simulink model "LQR_nonlinear_sim"  (R2025b)
settings: Solver=VariableStepAuto  StartTime=0.0  StopTime=5  RelTol=1e-3
undefined symbols (not defined in the file): A, B, bb, C, D, dotphi_x_ref, dotphi_y_ref, ic, ic_xy, ic_xz, ic_yz, K, K_vert, K_xy, Kr, N_vert
settings Model: Creator=JPham  LastModifiedBy=JPham

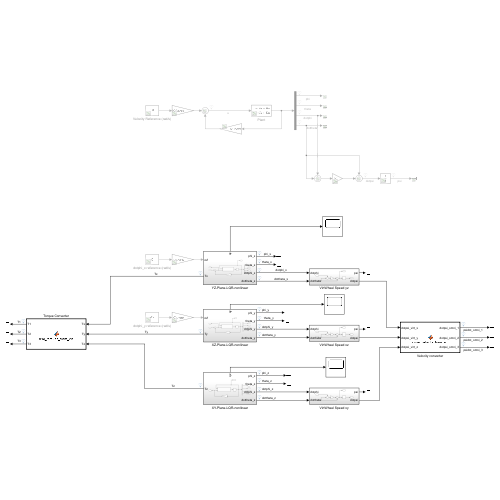
[thumbnail: Simulink's stored preview of the top-level diagram]
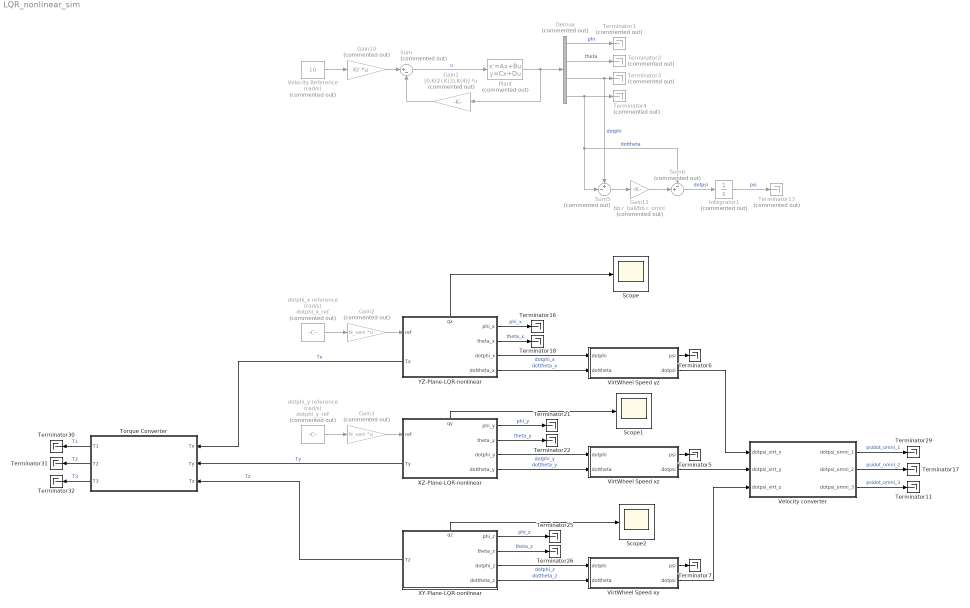
== system LQR_nonlinear_sim ==
  Demux : Demux  Commented=on
  Gain1 : Gain  Commented=on  Gain=[0,K(2),K(3),K(4)]  Multiplication=Matrix(K*u) (u vector)
  Gain10 : Gain  Commented=on  Gain=Kr  Multiplication=Matrix(K*u) (u vector)
  Gain11 : Gain  Commented=on  Gain=bb.r_ball/bb.r_omni
  Gain2 : Gain  Commented=on  Gain=N_vert  Multiplication=Matrix(K*u) (u vector)
  Gain3 : Gain  Commented=on  Gain=N_vert  Multiplication=Matrix(K*u) (u vector)
  Integrator1 : Integrator  Commented=on
  Plant : StateSpace  Commented=on  A=A  B=B  C=C  D=D  InitialCondition=ic  ContinuousStateAttributes={'phi', 'theta', 'dot_phi', 'dot_theta'}
  Scope : Scope
      settings: ActiveDisplayYMinimum=-1  ActiveDisplayYMaximum=1
  Scope1 : Scope
  Scope2 : Scope
      settings: DataLoggingVariableName=ScopeData2
  Sum : Sum  Commented=on  Inputs=|+-
  Sum5 : Sum  Commented=on  Inputs=+-|
  Sum6 : Sum  Commented=on  Inputs=-+|
  Terminator{1..4,13} (5 alike) : Terminator  Commented=on
  Terminator{5..7,11,16..18,21..22,25..26,29..32} (15 alike) : Terminator
  Torque Converter : MATLAB Function  TreatAsAtomicUnit=on
  Velocity Reference (rad/s) : Constant  Commented=on  Value=10
  Velocity converter : MATLAB Function  TreatAsAtomicUnit=on
  VirtWheel Speed xy : Subsystem
  VirtWheel Speed xz : Subsystem
  VirtWheel Speed yz : Subsystem
  XY-Plane-LQR-nonlinear : Subsystem
      settings: PortSchema="{\"entries\":[{\"content\":{\"sides\":[{\"content\":{\"connectorIds\":[\"Out6\"]},\"type\":\"ConnectorPlacement.EquallySpacedRectSide\",\"uuid\":\"02b8159c-179d-4bec-803c-aa283f49b9c0\"},{\"content\":{\"connectorIds\":[\"Out1\",\"Out2\",\"Out3\",\"Out4\"],\"side\":\"RIGHT\"},\"type\":\"ConnectorPlacement.EquallySpacedRectSide\",\"uuid\":\"3221cdc4-2dbb-4803-8373-e56db730aa56\"},{\"content\":{\"connectorIds\":[\"Out5\"],\"side\":\"TOP\"},\"type\":\"ConnectorPlacement.EquallySpacedRectSide\",\"uuid\":\"2bc7cb91-f8b8-434b-9ab0-3d8179530137\"}]},\"type\":\"ConnectorPlacement.EquallySpacedConnector\",\"uuid\":\"c9142ecd-3781-401c-ba0b-68be917d9976\"}],\"packageUris\":[\"http://schema.mathworks.com/mf0/Connector/R2020b\"],\"version\":\"1.0\"}"
  XZ-Plane-LQR-nonlinear : Subsystem
      settings: PortSchema="{\"entries\":[{\"content\":{\"sides\":[{\"content\":{\"connectorIds\":[\"In1\",\"Out6\"]},\"type\":\"ConnectorPlacement.EquallySpacedRectSide\",\"uuid\":\"02b8159c-179d-4bec-803c-aa283f49b9c0\"},{\"content\":{\"connectorIds\":[\"Out1\",\"Out2\",\"Out3\",\"Out4\"],\"side\":\"RIGHT\"},\"type\":\"ConnectorPlacement.EquallySpacedRectSide\",\"uuid\":\"3221cdc4-2dbb-4803-8373-e56db730aa56\"},{\"content\":{\"connectorIds\":[\"Out5\"],\"side\":\"TOP\"},\"type\":\"ConnectorPlacement.EquallySpacedRectSide\",\"uuid\":\"2bc7cb91-f8b8-434b-9ab0-3d8179530137\"}]},\"type\":\"ConnectorPlacement.EquallySpacedConnector\",\"uuid\":\"c9142ecd-3781-401c-ba0b-68be917d9976\"}],\"packageUris\":[\"http://schema.mathworks.com/mf0/Connector/R2020b\"],\"version\":\"1.0\"}"
  YZ-Plane-LQR-nonlinear : Subsystem
      settings: PortSchema="{\"entries\":[{\"content\":{\"sides\":[{\"content\":{\"connectorIds\":[\"In1\",\"Out6\"]},\"type\":\"ConnectorPlacement.EquallySpacedRectSide\",\"uuid\":\"02b8159c-179d-4bec-803c-aa283f49b9c0\"},{\"content\":{\"connectorIds\":[\"Out1\",\"Out2\",\"Out3\",\"Out4\"],\"side\":\"RIGHT\"},\"type\":\"ConnectorPlacement.EquallySpacedRectSide\",\"uuid\":\"3221cdc4-2dbb-4803-8373-e56db730aa56\"},{\"content\":{\"connectorIds\":[\"Out5\"],\"side\":\"TOP\"},\"type\":\"ConnectorPlacement.EquallySpacedRectSide\",\"uuid\":\"2bc7cb91-f8b8-434b-9ab0-3d8179530137\"}]},\"type\":\"ConnectorPlacement.EquallySpacedConnector\",\"uuid\":\"c9142ecd-3781-401c-ba0b-68be917d9976\"}],\"packageUris\":[\"http://schema.mathworks.com/mf0/Connector/R2020b\"],\"version\":\"1.0\"}"
  dotphi_x reference (rad/s) : Constant  Commented=on  Value=dotphi_x_ref
  dotphi_y reference (rad/s) : Constant  Commented=on  Value=dotphi_y_ref
  wires:
  Velocity Reference (rad/s)/1 -> Gain10/1
  Demux/1 -> Terminator1/1  "phi"
  Sum5/1 -> Gain11/1
  Sum6/1 -> Integrator1/1  "dotpsi"
  Demux/3 -> Sum5/1, Terminator3/1  "dotphi"
  Integrator1/1 -> Terminator13/1  "psi"
  Demux/2 -> Terminator2/1  "theta"
  Demux/4 -> Terminator4/1, Sum5/2, Sum6/1  "dottheta"
  Plant/1 -> Gain1/1, Demux/1
  Gain11/1 -> Sum6/2
  Gain10/1 -> Sum/1
  Sum/1 -> Plant/1  "u"
  Gain1/1 -> Sum/2
  VirtWheel Speed yz/2(dotpsi) -> Velocity converter/1(dotpsi_virt_x)
  VirtWheel Speed xy/2(dotpsi) -> Velocity converter/3(dotpsi_virt_z)
  Torque Converter/3(T3) -> Terminator32/1  "T3"
  Torque Converter/2(T2) -> Terminator31/1  "T2"
  Torque Converter/1(T1) -> Terminator30/1  "T1"
  VirtWheel Speed xz/2(dotpsi) -> Velocity converter/2(dotpsi_virt_y)
  VirtWheel Speed xz/1(psi) -> Terminator5/1
  VirtWheel Speed yz/1(psi) -> Terminator6/1
  VirtWheel Speed xy/1(psi) -> Terminator7/1
  YZ-Plane-LQR-nonlinear/6(Tx) -> Torque Converter/1(Tx)  "Tx"
  XZ-Plane-LQR-nonlinear/6(Ty) -> Torque Converter/2(Ty)  "Ty"
  XY-Plane-LQR-nonlinear/6(Tz) -> Torque Converter/3(Tz)  "Tz"
  YZ-Plane-LQR-nonlinear/3(dotphi_x) -> VirtWheel Speed yz/1(dotphi)  "dotphi_x"
  YZ-Plane-LQR-nonlinear/4(dottheta_x) -> VirtWheel Speed yz/2(dottheta)  "dottheta_x"
  YZ-Plane-LQR-nonlinear/2(theta_x) -> Terminator18/1  "theta_x"
  YZ-Plane-LQR-nonlinear/1(phi_x) -> Terminator16/1  "phi_x"
  XZ-Plane-LQR-nonlinear/4(dottheta_y) -> VirtWheel Speed xz/2(dottheta)  "dottheta_y"
  XZ-Plane-LQR-nonlinear/1(phi_y) -> Terminator21/1  "phi_y"
  XZ-Plane-LQR-nonlinear/2(theta_y) -> Terminator22/1  "theta_y"
  XZ-Plane-LQR-nonlinear/3(dotphi_y) -> VirtWheel Speed xz/1(dotphi)  "dotphi_y"
  XY-Plane-LQR-nonlinear/4(dottheta_z) -> VirtWheel Speed xy/2(dottheta)  "dottheta_z"
  XY-Plane-LQR-nonlinear/1(phi_z) -> Terminator25/1  "phi_z"
  XY-Plane-LQR-nonlinear/2(theta_z) -> Terminator26/1  "theta_z"
  XY-Plane-LQR-nonlinear/3(dotphi_z) -> VirtWheel Speed xy/1(dotphi)  "dotphi_z"
  dotphi_x reference (rad/s)/1 -> Gain2/1
  Gain2/1 -> YZ-Plane-LQR-nonlinear/1(ref)
  dotphi_y reference (rad/s)/1 -> Gain3/1
  Gain3/1 -> XZ-Plane-LQR-nonlinear/1(ref)
  Velocity converter/2(dotpsi_omni_2) -> Terminator17/1  "psidot_omni_2"
  Velocity converter/1(dotpsi_omni_1) -> Terminator29/1  "psidot_omni_1"
  Velocity converter/3(dotpsi_omni_3) -> Terminator11/1  "psidot_omni_3"
  YZ-Plane-LQR-nonlinear/5(qx) -> Scope/1
  XZ-Plane-LQR-nonlinear/5(qy) -> Scope1/1
  XY-Plane-LQR-nonlinear/5(qz) -> Scope2/1

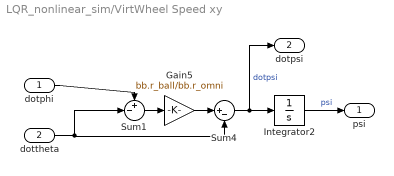
== system LQR_nonlinear_sim/VirtWheel Speed xy ==
  dotphi : Inport
  dottheta : Inport  Port=2
  Gain5 : Gain  Gain=bb.r_ball/bb.r_omni
  Integrator2 : Integrator
  Sum1 : Sum  Inputs=+-|
  Sum4 : Sum  Inputs=|+-
  psi : Outport
  dotpsi : Outport  Port=2
  wires:
  Sum1/1 -> Gain5/1
  dotphi/1 -> Sum1/1
  Integrator2/1 -> psi/1  "psi"
  Sum4/1 -> Integrator2/1, dotpsi/1  "dotpsi"
  dottheta/1 -> Sum4/2, Sum1/2
  Gain5/1 -> Sum4/1

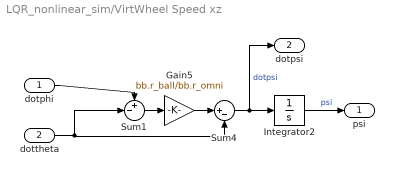
== system LQR_nonlinear_sim/VirtWheel Speed xz ==
  dotphi : Inport
  dottheta : Inport  Port=2
  Gain5 : Gain  Gain=bb.r_ball/bb.r_omni
  Integrator2 : Integrator
  Sum1 : Sum  Inputs=+-|
  Sum4 : Sum  Inputs=|+-
  psi : Outport
  dotpsi : Outport  Port=2
  wires:
  Gain5/1 -> Sum4/1
  dottheta/1 -> Sum1/2, Sum4/2
  Sum4/1 -> dotpsi/1, Integrator2/1  "dotpsi"
  Integrator2/1 -> psi/1  "psi"
  dotphi/1 -> Sum1/1
  Sum1/1 -> Gain5/1

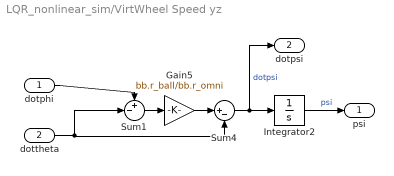
== system LQR_nonlinear_sim/VirtWheel Speed yz ==
  dotphi : Inport
  dottheta : Inport  Port=2
  Gain5 : Gain  Gain=bb.r_ball/bb.r_omni
  Integrator2 : Integrator
  Sum1 : Sum  Inputs=+-|
  Sum4 : Sum  Inputs=|+-
  psi : Outport
  dotpsi : Outport  Port=2
  wires:
  Sum1/1 -> Gain5/1
  dotphi/1 -> Sum1/1
  Integrator2/1 -> psi/1  "psi"
  Sum4/1 -> Integrator2/1, dotpsi/1  "dotpsi"
  dottheta/1 -> Sum4/2, Sum1/2
  Gain5/1 -> Sum4/1

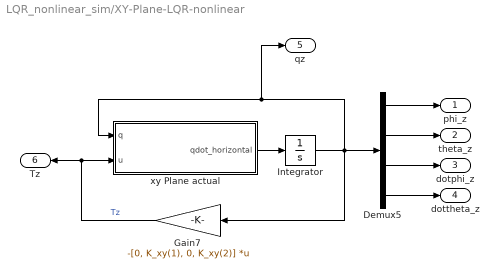
== system LQR_nonlinear_sim/XY-Plane-LQR-nonlinear ==
  Demux5 : Demux
  Gain7 : Gain  Gain=-[0, K_xy(1), 0, K_xy(2)]  Multiplication=Matrix(K*u) (u vector)
  Integrator : Integrator  InitialCondition=[0; ic_xy(1); 0; ic_xy(2)]
  xy Plane actual : MATLAB Function  TreatAsAtomicUnit=on
  phi_z : Outport
  theta_z : Outport  Port=2
  dotphi_z : Outport  Port=3
  dottheta_z : Outport  Port=4
  qz : Outport  Port=5
  Tz : Outport  Port=6
  wires:
  Demux5/1 -> phi_z/1
  Demux5/2 -> theta_z/1
  Integrator/1 -> qz/1, xy Plane actual/1(q), Gain7/1, Demux5/1
  Gain7/1 -> Tz/1, xy Plane actual/2(u)  "Tz"
  xy Plane actual/1(qdot_horizontal) -> Integrator/1
  Demux5/3 -> dotphi_z/1
  Demux5/4 -> dottheta_z/1

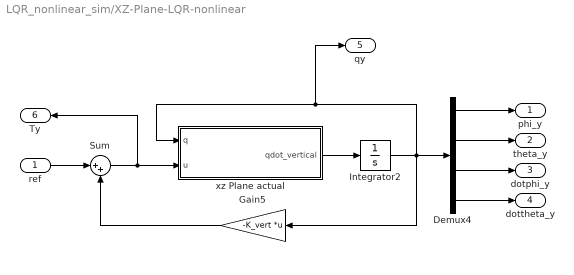
== system LQR_nonlinear_sim/XZ-Plane-LQR-nonlinear ==
  ref : Inport
  Demux4 : Demux
  Gain5 : Gain  Gain=-K_vert  Multiplication=Matrix(K*u) (u vector)
  Integrator2 : Integrator  InitialCondition=ic_xz  ContinuousStateAttributes='angle'
  Sum : Sum  Inputs=|++
  xz Plane actual : MATLAB Function  TreatAsAtomicUnit=on
  phi_y : Outport
  theta_y : Outport  Port=2
  dotphi_y : Outport  Port=3
  dottheta_y : Outport  Port=4
  qy : Outport  Port=5
  Ty : Outport  Port=6
  wires:
  Demux4/2 -> theta_y/1
  Integrator2/1 -> qy/1, xz Plane actual/1(q), Demux4/1, Gain5/1
  xz Plane actual/1(qdot_vertical) -> Integrator2/1
  Gain5/1 -> Sum/2
  Demux4/3 -> dotphi_y/1
  Demux4/1 -> phi_y/1
  Demux4/4 -> dottheta_y/1
  ref/1 -> Sum/1
  Sum/1 -> Ty/1, xz Plane actual/2(u)

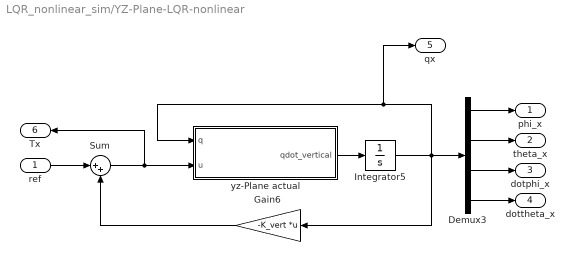
== system LQR_nonlinear_sim/YZ-Plane-LQR-nonlinear ==
  ref : Inport
  Demux3 : Demux
  Gain6 : Gain  Gain=-K_vert  Multiplication=Matrix(K*u) (u vector)
  Integrator5 : Integrator  InitialCondition=ic_yz  ContinuousStateAttributes='angle'
  Sum : Sum  Inputs=|++
  yz-Plane actual : MATLAB Function  TreatAsAtomicUnit=on
  phi_x : Outport
  theta_x : Outport  Port=2
  dotphi_x : Outport  Port=3
  dottheta_x : Outport  Port=4
  qx : Outport  Port=5
  Tx : Outport  Port=6
  wires:
  yz-Plane actual/1(qdot_vertical) -> Integrator5/1
  Integrator5/1 -> Gain6/1, Demux3/1, qx/1, yz-Plane actual/1(q)
  Demux3/3 -> dotphi_x/1
  Demux3/4 -> dottheta_x/1
  Gain6/1 -> Sum/2
  Demux3/2 -> theta_x/1
  Demux3/1 -> phi_x/1
  Sum/1 -> yz-Plane actual/2(u), Tx/1
  ref/1 -> Sum/1

== matlab function LQR_nonlinear_sim/YZ-Plane-LQR-nonlinear/yz-Plane actual ==
  data: q input; u input; qdot_vertical output
function qdot_vertical = f(q, u)
    % Define dimensions for code generation
    % x is 4x1 state: [phi; theta; phi_dot; theta_dot]
    % u is scalar torque (leave as constant for now)
    % p is the parameter structure, loaded into simulink in Model Explorer
    
    phi     = q(1); % phi
    theta   = q(2); % theta
    dotphi  = q(3); % phi_dot
    dottheta= q(4); % theta_dot
    
    p = params;
    % Aux Parameters
    m_tot = p.m_ball + p.m_body + p.m_virt;
    r_tot = p.r_ball + p.r_omni;
    gamma = p.l*p.m_body + (p.r_ball + p.r_omni)*p.m_virt;
    
    % M matrix
    M11 = m_tot * p.r_ball^2 + p.Theta_ball + (p.r_ball / p.r_omni)^2 * p.Theta_virt_vertical;
    M12 = -(p.r_ball / p.r_omni^2) * r_tot * p.Theta_virt_vertical + gamma * p.r_ball*cos(theta); 
    M22 = (r_tot^2 / p.r_omni^2) * p.Theta_virt_vertical + p.Theta_body_vertical + ...
           p.m_body * p.l^2 + p.m_virt * r_tot^2;
    M21 = M12;

    M = [M11, M12;
         M21, M22];
    
    % C vector
    Cvec = [ -p.r_ball*gamma*sin(theta)*dottheta^2; 
              0 ];
    % G vector
    Gvec = [ 0; 
            -p.g*sin(theta)*gamma ];
    % S vector (f_NP = S*u(t))
    S = [ p.r_ball / p.r_omni; -p.r_ball / p.r_omni ];
    
    % --- Dynamics Calculation ---
    F_np = S * u; 
    
    % Solve for qdd from M * qdd + C + G = F_np
    % qddot = M \ (F_np - C - G) = [theta_doubledot; phi_doubledot]
    qddot = M \ (F_np - Cvec - Gvec);
    
    % Assemble qdot_vertical
    qdot_vertical = [dotphi;
                     dottheta;
                     qddot(1);
                     qddot(2)];
end

== matlab function LQR_nonlinear_sim/XZ-Plane-LQR-nonlinear/xz Plane actual ==
  data: q input; u input; qdot_vertical output
function qdot_vertical = f(q, u)
    % Define dimensions for code generation
    % x is 4x1 state: [phi; theta; phi_dot; theta_dot]
    % u is scalar torque (leave as constant for now)
    % p is the parameter structure, loaded into simulink in Model Explorer
    
    phi     = q(1); % phi
    theta   = q(2); % theta
    dotphi  = q(3); % phi_dot
    dottheta= q(4); % theta_dot
    
    p = params;
    % Aux Parameters
    m_tot = p.m_ball + p.m_body + p.m_virt;
    r_tot = p.r_ball + p.r_omni;
    gamma = p.l*p.m_body + (p.r_ball + p.r_omni)*p.m_virt;
    
    % M matrix
    M11 = m_tot * p.r_ball^2 + p.Theta_ball + (p.r_ball / p.r_omni)^2 * p.Theta_virt_vertical;
    M12 = -(p.r_ball / p.r_omni^2) * r_tot * p.Theta_virt_vertical + gamma * p.r_ball*cos(theta); 
    M22 = (r_tot^2 / p.r_omni^2) * p.Theta_virt_vertical + p.Theta_body_vertical + ...
           p.m_body * p.l^2 + p.m_virt * r_tot^2;
    M21 = M12;

    M = [M11, M12;
         M21, M22];
    
    % C vector
    Cvec = [ -p.r_ball*gamma*sin(theta)*dottheta^2; 
              0 ];
    % G vector
    Gvec = [ 0; 
            -p.g*sin(theta)*gamma ];
    % S vector (f_NP = S*u(t))
    S = [ p.r_ball / p.r_omni; -p.r_ball / p.r_omni ];
    
    % --- Dynamics Calculation ---
    F_np = S * u; 
    
    % Solve for qdd from M * qdd + C + G = F_np
    % qddot = M \ (F_np - C - G) = [theta_doubledot; phi_doubledot]
    qddot = M \ (F_np - Cvec - Gvec);
    
    % Assemble qdot_vertical
    qdot_vertical = [dotphi;
                     dottheta;
                     qddot(1);
                     qddot(2)];
end

== matlab function LQR_nonlinear_sim/XY-Plane-LQR-nonlinear/xy Plane actual ==
  data: q input; u input; qdot_horizontal output
function qdot_horizontal = f(q, u)
    % Define dimensions for code generation
    % x is 4x1 state: [phi; theta; phi_dot; theta_dot]
    % u is scalar torque (leave as constant for now)
    % p is the parameter structure, loaded into simulink in Model Explorer
    
    phi     = q(1); % phi
    theta   = q(2); % theta
    dotphi  = q(3); % phi_dot
    dottheta= q(4); % theta_dot
    
    p = params;
    % Aux Parameters
    m_tot = p.m_ball + p.m_body + p.m_virt;
    r_tot = p.r_ball + p.r_omni;
    gamma = p.l*p.m_body + (p.r_ball + p.r_omni)*p.m_virt;
    
    T_f = ((p.r_ball*p.r_omni*p.Theta_body_xy*sin(p.alpha))...
        /((p.r_omni)^2*p.Theta_body_xy+(p.r_ball)^2*p.Theta_virt_xy*(sin(p.alpha))^2))*u;
    ddotphi = 0;
    ddottheta = -(p.r_ball*sin(p.alpha))*(p.r_ball*p.Theta_virt_xy*sin(p.alpha)+p.r_omni*p.Theta_ball)*T_f...
        /((p.r_omni)^2*p.Theta_body_xy*p.Theta_ball+(p.r_ball)^2*(p.Theta_body_xy+p.Theta_ball)*p.Theta_virt_xy*(sin(p.alpha))^2);
    
    % Assemble qdot_vertical
    qdot_horizontal = [dotphi;
                     dottheta;
                     ddotphi;
                     ddottheta];
end

== matlab function LQR_nonlinear_sim/Torque Converter ==
  data: Tx input; Ty input; T1 output; Tz input; T2 output; T3 output
function [T1, T2, T3] = real_torques_from_virt(Tx, Ty, Tz)
alpha = params().alpha;
beta  = params().beta;

cosa = cos(alpha);
cb = cos(beta);
sb = sin(beta);

T1 = (1/3) * ( ...
      Tz + (2/cosa) * (Tx*cb - Ty*sb) );

T2 = (1/3) * ( ...
      Tz + (1/cosa) * ( sb*(-sqrt(3)*Tx + Ty) ...
                      - cb*( Tx + sqrt(3)*Ty ) ) );

T3 = (1/3) * ( ...
      Tz + (1/cosa) * ( sb*( sqrt(3)*Tx + Ty) ...
                      + cb*(-Tx + sqrt(3)*Ty ) ) );

end

== matlab function LQR_nonlinear_sim/Velocity converter ==
  data: dotpsi_virt_x input; dotpsi_virt_y input; dotpsi_omni_1 output; dotpsi_virt_z input; dotpsi_omni_2 output; dotpsi_omni_3 output
% This function convert the velocity of the virtual wheels
% from three planes to the velocity of the omniwheels.
% for beta = 0

function [dotpsi_omni_1, dotpsi_omni_2, dotpsi_omni_3] = ...
    omni_velocity_from_virt(dotpsi_virt_x, dotpsi_virt_y, dotpsi_virt_z)
bb = params();
rads_to_rpm = 30/pi;

dotpsi_omni_1 = (dotpsi_virt_x * cos(bb.alpha) ...
    + dotpsi_virt_z*sin(bb.alpha))*rads_to_rpm;
dotpsi_omni_2 = (-0.5 * dotpsi_virt_x * cos(bb.alpha) ...
    - sqrt(3)*dotpsi_virt_y*cos(bb.alpha)/2 ...
    + dotpsi_virt_z*sin(bb.alpha))* rads_to_rpm;
dotpsi_omni_3 = (-0.5 * dotpsi_virt_x * cos(bb.alpha) ...
    + sqrt(3)*dotpsi_virt_y*cos(bb.alpha)/2 ...
    + dotpsi_virt_z*sin(bb.alpha))* rads_to_rpm;
end
